simulink model "Appl_VentAdj_CtrlModel"  (R2018b)
settings: configuration reference "CodeConfig_10_ms" (kept outside this file)
undefined symbols (not defined in the file): D_VENT_LVL_1_PRECENT, D_VENT_LVL_2_PRECENT, D_VENT_LVL_3_PRECENT, FALSE, TRUE
libraries: DareLib x72, simulink x1
(part 1 of 4)
settings Model: Creator=Administrator  LastModifiedBy=Administrator
settings ConfigSetRef: SourceLocation=Base Workspace

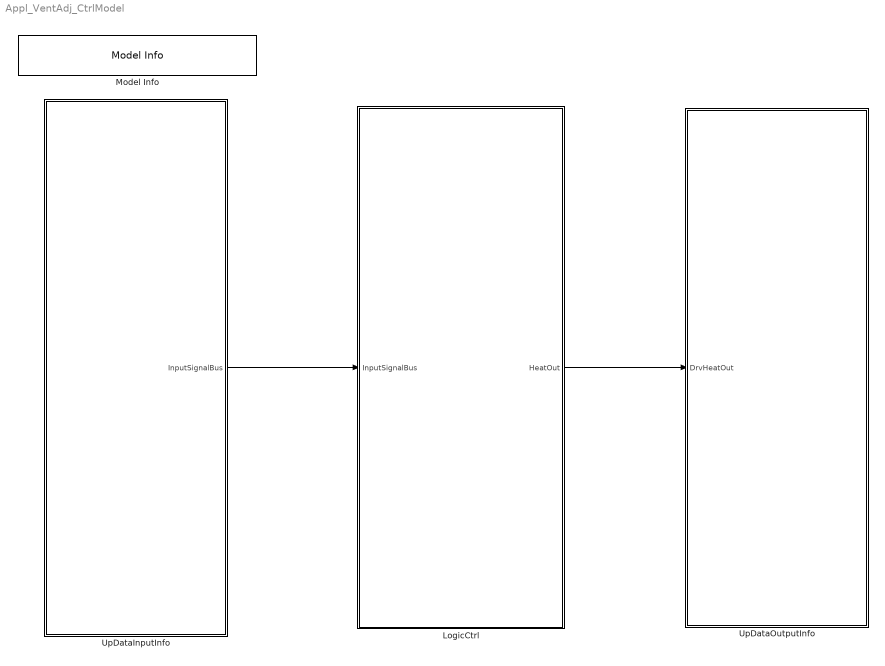
== system Appl_VentAdj_CtrlModel ==
  LogicCtrl : Subsystem  Priority=2  TreatAsAtomicUnit=on
      settings: RTWSystemCode=Nonreusable function  RTWFcnNameOpts=Use subsystem name
  Model Info : simulink/Model-Wide Utilities/Model Info  Frame=on  DisplayStringWithTags=Version：%<ModelVersion>  HorizontalTextAlignment=Center  LeftAlignmentValue=0.5
  UpDataInputInfo : Subsystem  Priority=1  TreatAsAtomicUnit=on
      settings: RTWSystemCode=Nonreusable function  RTWFcnNameOpts=Use subsystem name
  UpDataOutputInfo : Subsystem  Priority=3  TreatAsAtomicUnit=on
      settings: RTWSystemCode=Nonreusable function  RTWFcnNameOpts=Use subsystem name
  wires:
  LogicCtrl/1(HeatOut) -> UpDataOutputInfo/1(DrvHeatOut)
  UpDataInputInfo/1(InputSignalBus) -> LogicCtrl/1(InputSignalBus)

== system Appl_VentAdj_CtrlModel/LogicCtrl ==
  InputSignalBus : Inport
  Bus Selector : BusSelector  OutputSignals=VentRunMaxTime,HeatValid,Rte_SignalBUs.VentAdj_D_SimuIndex_DRVent,Rte_SignalBUs.VentAdj_D_SimuIndex_PAVent,Rte_SignalBUs.VentAdj_D_SimuIndex_ThirdVent,Rte_SignalBUs.VentAdj_CarType,Rte_SignalBUs.VentAdj_RemoteModeFlag,Rte_SignalBUs.VentAdj_EngineRunFlag,Rte_SignalBUs.VentAdj_DriverCmdFaultSts,Rte_SignalBUs.VentAdj_PasCmdFaultSts,Rte_SignalBUs.VentAdj_ThirdCmdFaultSts,Rte_SignalBUs.VentAdj_PowerMode,Rte_SignalBUs.VentAdj_DriverEnableConfig,Rte_SignalBUs.VentAdj_DriverHMI_VentMessage,Rte_SignalBUs.VentAdj_DriverTbox_VentMessage,Rte_SignalBUs.VentAdj_PassengerEnableConfig,Rte_SignalBUs.VentAdj_PassengerHMI_VentMessage,Rte_SignalBUs.VentAdj_PassengerTbox_VentMessage,Rte_SignalBUs.VentAdj_ThirdEnableConfig,Rte_SignalBUs.VentAdj_ThirdHMI_VentMessage,Rte_SignalBUs.VentAdj_ThirdTbox_VentMessage,Rte_SignalBUs.VentAdj_DriverDiagCmd,Rte_SignalBUs.VentAdj_PassengerDiagCmd,Rte_SignalBUs.VentAdj_ThirdDiagCmd,Rte_SignalBUs.VentAdj_TimeOutPrm,Rte_SignalBUs.VentAdj_RunMaxTime,Rte_SignalBUs.VentAdj_VoltMode,Rte_SignalBUs.VentAdj_RecoverDefaultFlag,Rte_SignalBUs.VentAdj_Driver_HMI_HeatMsg,Rte_SignalBUs.VentAdj_Driver_Tbox_HeatMsg,Rte_SignalBUs.VentAdj_Passenger_HMI_HeatMsg,Rte_SignalBUs.VentAdj_Passenger_Tbox_HeatMsg,Rte_SignalBUs.VentAdj_Third_HMI_HeatMsg,Rte_SignalBUs.VentAdj_Third_Tbox_HeatMsg,Rte_SignalBUs.VentAdj_DrVentStopReason,Rte_SignalBUs.VentAdj_PaVentStopReason,Rte_SignalBUs.VentAdj_ThirdVentStopReason,Rte_SignalBUs.VentAdj_VentMsgLostFlag,VentMessage,Rte_SignalBUs.VentAdj_CanDrvVentLvl,Rte_SignalBUs.VentAdj_CanPasVentLvl,Rte_SignalBUs.VentAdj_CanThirdVentLvl,Rte_SignalBUs.VentAdj_DriverCmdFaultSts4DTC,Rte_SignalBUs.VentAdj_PasCmdFaultSts4DTC,Rte_SignalBUs.VentAdj_ThirdCmdFaultSts4DTC,ComPCSatisfiedFlag,VentEnable
  LocalAdjustCtrl : Subsystem  Description=逻辑处理
      settings: AttributesFormatString=%<Description>
  MainVent_OutputLvlSts : BusCreator  Inputs=18
  HeatOut : Outport
  wires:
  InputSignalBus/1 -> Bus Selector/1  "InputSignalBus"
  MainVent_OutputLvlSts/1 -> HeatOut/1
  Bus Selector/1 -> LocalAdjustCtrl/1(VentRunMaxTime)  "<VentRunMaxTime>"
  Bus Selector/2 -> LocalAdjustCtrl/2(HeatValid)  "<HeatValid>"
  Bus Selector/3 -> LocalAdjustCtrl/3(VentAdj_D_SimuIndex_DRVent)  "<VentAdj_D_SimuIndex_DRVent>"
  Bus Selector/4 -> LocalAdjustCtrl/4(VentAdj_D_SimuIndex_PAVent)  "<VentAdj_D_SimuIndex_PAVent>"
  Bus Selector/5 -> LocalAdjustCtrl/5(VentAdj_D_SimuIndex_ThirdVent)  "<VentAdj_D_SimuIndex_ThirdVent>"
  Bus Selector/6 -> LocalAdjustCtrl/6(VentAdj_CarType)  "<VentAdj_CarType>"
  Bus Selector/7 -> LocalAdjustCtrl/7(VentAdj_RemoteModeFlag)  "<VentAdj_RemoteModeFlag>"
  Bus Selector/8 -> LocalAdjustCtrl/8(VentAdj_EngineRunFlag)  "<VentAdj_EngineRunFlag>"
  Bus Selector/9 -> LocalAdjustCtrl/9(VentAdj_DriverCmdFaultSts)  "<VentAdj_DriverCmdFaultSts>"
  Bus Selector/10 -> LocalAdjustCtrl/10(VentAdj_PasCmdFaultSts)  "<VentAdj_PasCmdFaultSts>"
  Bus Selector/11 -> LocalAdjustCtrl/11(VentAdj_ThirdCmdFaultSts)  "<VentAdj_ThirdCmdFaultSts>"
  Bus Selector/12 -> LocalAdjustCtrl/12(VentAdj_PowerMode)  "<VentAdj_PowerMode>"
  Bus Selector/13 -> LocalAdjustCtrl/13(VentAdj_DriverEnableConfig)  "<VentAdj_DriverEnableConfig>"
  Bus Selector/14 -> LocalAdjustCtrl/14(VentAdj_DriverHMI_VentMessage)  "<VentAdj_DriverHMI_VentMessage>"
  Bus Selector/15 -> LocalAdjustCtrl/15(VentAdj_DriverTbox_VentMessage)  "<VentAdj_DriverTbox_VentMessage>"
  Bus Selector/16 -> LocalAdjustCtrl/16(VentAdj_PassengerEnableConfig)  "<VentAdj_PassengerEnableConfig>"
  Bus Selector/17 -> LocalAdjustCtrl/17(VentAdj_PassengerHMI_VentMessage)  "<VentAdj_PassengerHMI_VentMessage>"
  Bus Selector/18 -> LocalAdjustCtrl/18(VentAdj_PassengerTbox_VentMessage)  "<VentAdj_PassengerTbox_VentMessage>"
  Bus Selector/19 -> LocalAdjustCtrl/19(VentAdj_ThirdEnableConfig)  "<VentAdj_ThirdEnableConfig>"
  Bus Selector/20 -> LocalAdjustCtrl/20(VentAdj_ThirdHMI_VentMessage)  "<VentAdj_ThirdHMI_VentMessage>"
  Bus Selector/21 -> LocalAdjustCtrl/21(VentAdj_ThirdTbox_VentMessage)  "<VentAdj_ThirdTbox_VentMessage>"
  Bus Selector/22 -> LocalAdjustCtrl/22(VentAdj_DriverDiagCmd)  "<VentAdj_DriverDiagCmd>"
  Bus Selector/23 -> LocalAdjustCtrl/23(VentAdj_PassengerDiagCmd)  "<VentAdj_PassengerDiagCmd>"
  Bus Selector/24 -> LocalAdjustCtrl/24(VentAdj_ThirdDiagCmd)  "<VentAdj_ThirdDiagCmd>"
  Bus Selector/25 -> LocalAdjustCtrl/25(VentAdj_TimeOutPrm)  "<VentAdj_TimeOutPrm>"
  Bus Selector/26 -> LocalAdjustCtrl/26(VentAdj_RunMaxTime)  "<VentAdj_RunMaxTime>"
  Bus Selector/27 -> LocalAdjustCtrl/27(VentAdj_VoltMode)  "<VentAdj_VoltMode>"
  Bus Selector/28 -> LocalAdjustCtrl/28(VentAdj_RecoverDefaultFlag)  "<VentAdj_RecoverDefaultFlag>"
  Bus Selector/29 -> LocalAdjustCtrl/29(VentAdj_Driver_HMI_HeatMsg)  "<VentAdj_Driver_HMI_HeatMsg>"
  Bus Selector/30 -> LocalAdjustCtrl/30(VentAdj_Driver_Tbox_HeatMsg)  "<VentAdj_Driver_Tbox_HeatMsg>"
  Bus Selector/31 -> LocalAdjustCtrl/31(VentAdj_Passenger_HMI_HeatMsg)  "<VentAdj_Passenger_HMI_HeatMsg>"
  Bus Selector/32 -> LocalAdjustCtrl/32(VentAdj_Passenger_Tbox_HeatMsg)  "<VentAdj_Passenger_Tbox_HeatMsg>"
  Bus Selector/33 -> LocalAdjustCtrl/33(VentAdj_Third_HMI_HeatMsg)  "<VentAdj_Third_HMI_HeatMsg>"
  Bus Selector/34 -> LocalAdjustCtrl/34(VentAdj_Third_Tbox_HeatMsg)  "<VentAdj_Third_Tbox_HeatMsg>"
  Bus Selector/35 -> LocalAdjustCtrl/35(VentAdj_DrVentStopReason)  "<VentAdj_DrVentStopReason>"
  Bus Selector/36 -> LocalAdjustCtrl/36(VentAdj_PaVentStopReason)  "<VentAdj_PaVentStopReason>"
  Bus Selector/37 -> LocalAdjustCtrl/37(VentAdj_ThirdVentStopReason)  "<VentAdj_ThirdVentStopReason>"
  Bus Selector/38 -> LocalAdjustCtrl/38(VentAdj_VentMsgLostFlag)  "<VentAdj_VentMsgLostFlag>"
  LocalAdjustCtrl/1(VentAdj_DrVentStopReasonOut) -> MainVent_OutputLvlSts/1
  LocalAdjustCtrl/2(VentAdj_PaVentStopReasonOut) -> MainVent_OutputLvlSts/2
  LocalAdjustCtrl/3(VentAdj_ThirdVentStopReasonOut) -> MainVent_OutputLvlSts/3
  LocalAdjustCtrl/4(VentAdj_DrVentTypeOut) -> MainVent_OutputLvlSts/4
  LocalAdjustCtrl/5(VentAdj_PaVentTypeOut) -> MainVent_OutputLvlSts/5
  LocalAdjustCtrl/6(VentAdj_ThirdVentTypeOut) -> MainVent_OutputLvlSts/6
  LocalAdjustCtrl/7(HeatAdj_DRVentOut) -> MainVent_OutputLvlSts/7
  LocalAdjustCtrl/8(HeatAdj_PAVentOut) -> MainVent_OutputLvlSts/8
  LocalAdjustCtrl/9(HeatAdj_ThirdVentOut) -> MainVent_OutputLvlSts/9
  LocalAdjustCtrl/10(HeatAdj_DRVentDuty) -> MainVent_OutputLvlSts/10
  LocalAdjustCtrl/11(HeatAdj_PAVentDuty) -> MainVent_OutputLvlSts/11
  LocalAdjustCtrl/12(HeatAdj_ThirdVentDuty) -> MainVent_OutputLvlSts/12
  LocalAdjustCtrl/13(HeatAdj_DrRunStateOut) -> MainVent_OutputLvlSts/13
  LocalAdjustCtrl/14(HeatAdj_PaRunStateOut) -> MainVent_OutputLvlSts/14
  LocalAdjustCtrl/15(HeatAdj_3rdRunStateOut) -> MainVent_OutputLvlSts/15
  Bus Selector/39 -> LocalAdjustCtrl/39(VentMessage)  "<VentMessage>"
  LocalAdjustCtrl/16(DiagDrVentLevel) -> MainVent_OutputLvlSts/16
  LocalAdjustCtrl/17(DiagPaVentLevel) -> MainVent_OutputLvlSts/17
  LocalAdjustCtrl/18(Diag3rdVentLevel) -> MainVent_OutputLvlSts/18
  Bus Selector/40 -> LocalAdjustCtrl/40(VentAdj_CanDrvVentLvl)  "<VentAdj_CanDrvVentLvl>"
  Bus Selector/41 -> LocalAdjustCtrl/41(VentAdj_CanPasVentLvl)  "<VentAdj_CanPasVentLvl>"
  Bus Selector/42 -> LocalAdjustCtrl/42(VentAdj_CanThirdVentLvl)  "<VentAdj_CanThirdVentLvl>"
  Bus Selector/43 -> LocalAdjustCtrl/43(VentAdj_DriverCmdFaultSts4DTC)  "<VentAdj_DriverCmdFaultSts4DTC>"
  Bus Selector/44 -> LocalAdjustCtrl/44(VentAdj_PasCmdFaultSts4DTC)  "<VentAdj_PasCmdFaultSts4DTC>"
  Bus Selector/45 -> LocalAdjustCtrl/45(VentAdj_ThirdCmdFaultSts4DTC)  "<VentAdj_ThirdCmdFaultSts4DTC>"
  Bus Selector/46 -> LocalAdjustCtrl/46(ComPCSatisfiedFlag)  "<ComPCSatisfiedFlag>"
  Bus Selector/47 -> LocalAdjustCtrl/47(VentEnable)  "<VentEnable>"

== system Appl_VentAdj_CtrlModel/UpDataInputInfo ==
  InputSignalProcess : Subsystem  Description=数据处理
      settings: AttributesFormatString=%<Description>  RTWSystemCode=Nonreusable function  RTWFcnNameOpts=Use subsystem name
  RTE : Subsystem  Description=接口自动生成  TreatAsAtomicUnit=on
      settings: AttributesFormatString=%<Description>  RTWSystemCode=Nonreusable function  RTWFcnNameOpts=Use subsystem name
  InputSignalBus : Outport
  wires:
  RTE/1(RTE_Signal) -> InputSignalProcess/1(Rte_SignalBUs)
  InputSignalProcess/1(InputSignalBus) -> InputSignalBus/1

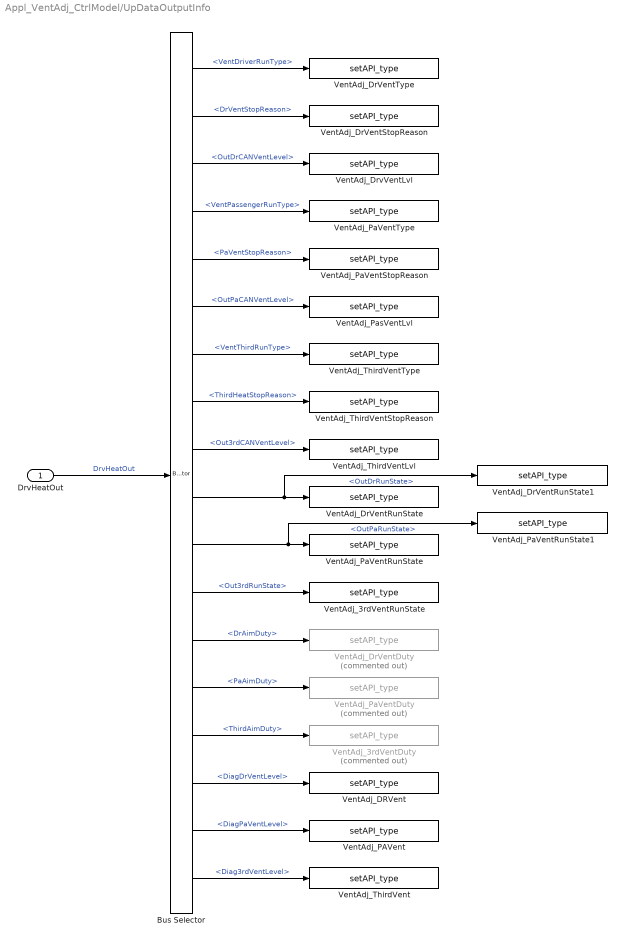
== system Appl_VentAdj_CtrlModel/UpDataOutputInfo ==
  DrvHeatOut : Inport
  Bus Selector : BusSelector  OutputSignals=VentDriverRunType,DrVentStopReason,OutDrCANVentLevel,VentPassengerRunType,PaVentStopReason,OutPaCANVentLevel,VentThirdRunType,ThirdHeatStopReason,Out3rdCANVentLevel,OutDrRunState,OutPaRunState,Out3rdRunState,DrAimDuty,PaAimDuty,ThirdAimDuty,DiagDrVentLevel,DiagPaVentLevel,Diag3rdVentLevel
  VentAdj_3rdVentDuty : DareLib/Dare/setAPI_type  Commented=on  g_funcname=Ecual_PWM_ChannelSetDuty  g_param=""  g_type=uint8  g_size=-1
      settings: AttributesFormatString=%<g_funcname>  SourceProductName=Dare Library
  VentAdj_3rdVentRunState : DareLib/Dare/setAPI_type  g_funcname=Rte_SetVfb_ThirdVentRunState  g_param=""  g_type=uint8  g_size=-1
      settings: AttributesFormatString=%<g_funcname>  SourceProductName=Dare Library
  VentAdj_DRVent : DareLib/Dare/setAPI_type  g_funcname=Rte_SetVfb_DrVent  g_param=""  g_type=uint8  g_enum=enVentLvlSts  g_size=-1
      settings: AttributesFormatString=%<g_funcname>  SourceProductName=Dare Library
  VentAdj_DrVentDuty : DareLib/Dare/setAPI_type  Commented=on  g_funcname=Ecual_PWM_ChannelSetDuty  g_param=""  g_type=uint8  g_size=-1
      settings: AttributesFormatString=%<g_funcname>  SourceProductName=Dare Library
  VentAdj_DrVentRunState : DareLib/Dare/setAPI_type  g_funcname=Rte_SetVfb_DrVentRunState  g_param=""  g_type=uint8  g_size=-1
      settings: AttributesFormatString=%<g_funcname>  SourceProductName=Dare Library
  VentAdj_DrVentRunState1 : DareLib/Dare/setAPI_type  g_funcname=Ecual_CanSetDrvVentSts  g_param=""  g_type=uint8  g_size=-1
      settings: AttributesFormatString=%<g_funcname>  SourceProductName=Dare Library
  VentAdj_DrVentStopReason : DareLib/Dare/setAPI_type  g_funcname=Rte_SetVfb_DrVentStopReason  g_param=""  g_type=uint8  g_enum=enVentStopReason  g_size=-1
      settings: AttributesFormatString=%<g_funcname>  SourceProductName=Dare Library
  VentAdj_DrVentType : DareLib/Dare/setAPI_type  g_funcname=Rte_SetVfb_DrVentType  g_param=""  g_type=uint8  g_enum=enVentType  g_size=-1
      settings: AttributesFormatString=%<g_funcname>  SourceProductName=Dare Library
  VentAdj_DrvVentLvl : DareLib/Dare/setAPI_type  g_funcname=Ecual_CanSetDrvVentLvl  g_param=""  g_type=uint8  g_enum=enVentLvlSts  g_size=-1
      settings: AttributesFormatString=%<g_funcname>  SourceProductName=Dare Library
  VentAdj_PAVent : DareLib/Dare/setAPI_type  g_funcname=Rte_SetVfb_PaVent  g_param=""  g_type=uint8  g_enum=enVentLvlSts  g_size=-1
      settings: AttributesFormatString=%<g_funcname>  SourceProductName=Dare Library
  VentAdj_PaVentDuty : DareLib/Dare/setAPI_type  Commented=on  g_funcname=Ecual_PWM_ChannelSetDuty  g_param=""  g_type=uint8  g_size=-1
      settings: AttributesFormatString=%<g_funcname>  SourceProductName=Dare Library
  VentAdj_PaVentRunState : DareLib/Dare/setAPI_type  g_funcname=Rte_SetVfb_PaVentRunState  g_param=""  g_type=uint8  g_size=-1
      settings: AttributesFormatString=%<g_funcname>  SourceProductName=Dare Library
  VentAdj_PaVentRunState1 : DareLib/Dare/setAPI_type  g_funcname=Ecual_CanSetPasVentSts  g_param=""  g_type=uint8  g_size=-1
      settings: AttributesFormatString=%<g_funcname>  SourceProductName=Dare Library
  VentAdj_PaVentStopReason : DareLib/Dare/setAPI_type  g_funcname=Rte_SetVfb_PaVentStopReason  g_param=""  g_type=uint8  g_enum=enVentStopReason  g_size=-1
      settings: AttributesFormatString=%<g_funcname>  SourceProductName=Dare Library
  VentAdj_PaVentType : DareLib/Dare/setAPI_type  g_funcname=Rte_SetVfb_PaVentType  g_param=""  g_type=uint8  g_enum=enVentType  g_size=-1
      settings: AttributesFormatString=%<g_funcname>  SourceProductName=Dare Library
  VentAdj_PasVentLvl : DareLib/Dare/setAPI_type  g_funcname=Ecual_CanSetPasVentLvl  g_param=""  g_type=uint8  g_enum=enVentLvlSts  g_size=-1
      settings: AttributesFormatString=%<g_funcname>  SourceProductName=Dare Library
  VentAdj_ThirdVent : DareLib/Dare/setAPI_type  g_funcname=Rte_SetVfb_ThirdVent  g_param=""  g_type=uint8  g_enum=enVentLvlSts  g_size=-1
      settings: AttributesFormatString=%<g_funcname>  SourceProductName=Dare Library
  VentAdj_ThirdVentLvl : DareLib/Dare/setAPI_type  g_funcname=Ecual_CanSetThirdVentLvl  g_param=""  g_type=uint8  g_enum=enVentLvlSts  g_size=-1
      settings: AttributesFormatString=%<g_funcname>  SourceProductName=Dare Library
  VentAdj_ThirdVentStopReason : DareLib/Dare/setAPI_type  g_funcname=Rte_SetVfb_ThirdVentStopReason  g_param=""  g_type=uint8  g_enum=enVentStopReason  g_size=-1
      settings: AttributesFormatString=%<g_funcname>  SourceProductName=Dare Library
  VentAdj_ThirdVentType : DareLib/Dare/setAPI_type  g_funcname=Rte_SetVfb_ThirdVentType  g_param=""  g_type=uint8  g_enum=enVentType  g_size=-1
      settings: AttributesFormatString=%<g_funcname>  SourceProductName=Dare Library
  wires:
  DrvHeatOut/1 -> Bus Selector/1  "DrvHeatOut"
  Bus Selector/1 -> VentAdj_DrVentType/1  "<VentDriverRunType>"
  Bus Selector/2 -> VentAdj_DrVentStopReason/1  "<DrVentStopReason>"
  Bus Selector/3 -> VentAdj_DrvVentLvl/1  "<OutDrCANVentLevel>"
  Bus Selector/6 -> VentAdj_PasVentLvl/1  "<OutPaCANVentLevel>"
  Bus Selector/5 -> VentAdj_PaVentStopReason/1  "<PaVentStopReason>"
  Bus Selector/4 -> VentAdj_PaVentType/1  "<VentPassengerRunType>"
  Bus Selector/9 -> VentAdj_ThirdVentLvl/1  "<Out3rdCANVentLevel>"
  Bus Selector/8 -> VentAdj_ThirdVentStopReason/1  "<ThirdHeatStopReason>"
  Bus Selector/7 -> VentAdj_ThirdVentType/1  "<VentThirdRunType>"
  Bus Selector/15 -> VentAdj_3rdVentDuty/1  "<ThirdAimDuty>"
  Bus Selector/14 -> VentAdj_PaVentDuty/1  "<PaAimDuty>"
  Bus Selector/13 -> VentAdj_DrVentDuty/1  "<DrAimDuty>"
  Bus Selector/12 -> VentAdj_3rdVentRunState/1  "<Out3rdRunState>"
  Bus Selector/11 -> VentAdj_PaVentRunState1/1, VentAdj_PaVentRunState/1  "<OutPaRunState>"
  Bus Selector/10 -> VentAdj_DrVentRunState1/1, VentAdj_DrVentRunState/1  "<OutDrRunState>"
  Bus Selector/16 -> VentAdj_DRVent/1  "<DiagDrVentLevel>"
  Bus Selector/17 -> VentAdj_PAVent/1  "<DiagPaVentLevel>"
  Bus Selector/18 -> VentAdj_ThirdVent/1  "<Diag3rdVentLevel>"

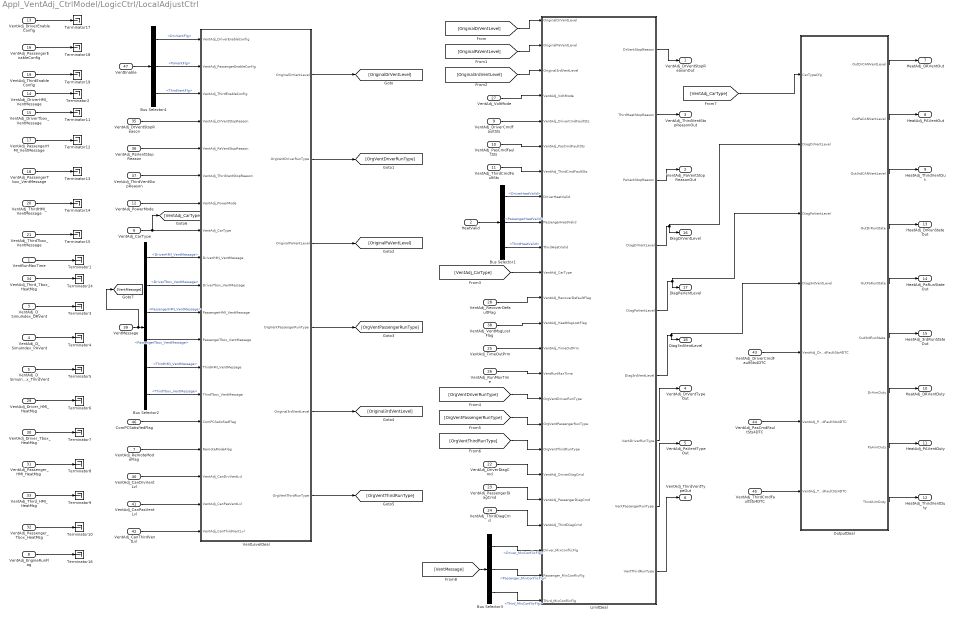
== system Appl_VentAdj_CtrlModel/LogicCtrl/LocalAdjustCtrl ==
  VentRunMaxTime : Inport
  HeatValid : Inport  Port=2
  VentAdj_D_SimuIndex_DRVent : Inport  Port=3
  VentAdj_D_SimuIndex_PAVent : Inport  Port=4
  VentAdj_D_SimuIndex_ThirdVent : Inport  Port=5
  VentAdj_CarType : Inport  Port=6
  VentAdj_RemoteModeFlag : Inport  Port=7
  VentAdj_EngineRunFlag : Inport  Port=8
  VentAdj_DriverCmdFaultSts : Inport  Port=9
  VentAdj_PasCmdFaultSts : Inport  Port=10
  VentAdj_ThirdCmdFaultSts : Inport  Port=11
  VentAdj_PowerMode : Inport  Port=12
  VentAdj_DriverEnableConfig : Inport  Port=13
  VentAdj_DriverHMI_VentMessage : Inport  Port=14
  VentAdj_DriverTbox_VentMessage : Inport  Port=15
  VentAdj_PassengerEnableConfig : Inport  Port=16
  VentAdj_PassengerHMI_VentMessage : Inport  Port=17
  VentAdj_PassengerTbox_VentMessage : Inport  Port=18
  VentAdj_ThirdEnableConfig : Inport  Port=19
  VentAdj_ThirdHMI_VentMessage : Inport  Port=20
  VentAdj_ThirdTbox_VentMessage : Inport  Port=21
  VentAdj_DriverDiagCmd : Inport  Port=22
  VentAdj_PassengerDiagCmd : Inport  Port=23
  VentAdj_ThirdDiagCmd : Inport  Port=24
  VentAdj_TimeOutPrm : Inport  Port=25
  VentAdj_RunMaxTime : Inport  Port=26
  VentAdj_VoltMode : Inport  Port=27
  VentAdj_RecoverDefaultFlag : Inport  Port=28
  VentAdj_Driver_HMI_HeatMsg : Inport  Port=29
  VentAdj_Driver_Tbox_HeatMsg : Inport  Port=30
  VentAdj_Passenger_HMI_HeatMsg : Inport  Port=31
  VentAdj_Passenger_Tbox_HeatMsg : Inport  Port=32
  VentAdj_Third_HMI_HeatMsg : Inport  Port=33
  VentAdj_Third_Tbox_HeatMsg : Inport  Port=34
  VentAdj_DrVentStopReason : Inport  Port=35
  VentAdj_PaVentStopReason : Inport  Port=36
  VentAdj_ThirdVentStopReason : Inport  Port=37
  VentAdj_VentMsgLostFlag : Inport  Port=38
  VentMessage : Inport  Port=39
  VentAdj_CanDrvVentLvl : Inport  Port=40
  VentAdj_CanPasVentLvl : Inport  Port=41
  VentAdj_CanThirdVentLvl : Inport  Port=42
  VentAdj_DriverCmdFaultSts4DTC : Inport  Port=43
  VentAdj_PasCmdFaultSts4DTC : Inport  Port=44
  VentAdj_ThirdCmdFaultSts4DTC : Inport  Port=45
  ComPCSatisfiedFlag : Inport  Port=46
  VentEnable : Inport  Port=47
  Bus Selector1 : BusSelector  OutputSignals=DriverHeatValid,PassengerHeatValid,ThirdHeatValid
  Bus Selector2 : BusSelector  OutputSignals=DriverHMI_VentMessage,DriverTbox_VentMessage,PassengerHMI_VentMessage,PassengerTbox_VentMessage,ThirdHMI_VentMessage,ThirdTbox_VentMessage
  Bus Selector3 : BusSelector  OutputSignals=Driver_MixConflicFlg,Passenger_MixConflicFlg,Third_MixConflicFlg
  Bus Selector4 : BusSelector  OutputSignals=DrvVentFlg,PaVentFlg,ThirdVentFlg
  LimitDeal : Stateflow chart  TreatAsAtomicUnit=on
  OutputDeal : Stateflow chart  TreatAsAtomicUnit=on
  Terminator{1..19,24} (20 alike) : Terminator
  VentLevelDeal : Stateflow chart  TreatAsAtomicUnit=on
  VentAdj_DrVentStopReasonOut : Outport
  VentAdj_PaVentStopReasonOut : Outport  Port=2
  VentAdj_ThirdVentStopReasonOut : Outport  Port=3
  VentAdj_DrVentTypeOut : Outport  Port=4
  VentAdj_PaVentTypeOut : Outport  Port=5
  VentAdj_ThirdVentTypeOut : Outport  Port=6
  HeatAdj_DRVentOut : Outport  Port=7
  HeatAdj_PAVentOut : Outport  Port=8
  HeatAdj_ThirdVentOut : Outport  Port=9
  HeatAdj_DRVentDuty : Outport  Port=10
  HeatAdj_PAVentDuty : Outport  Port=11
  HeatAdj_ThirdVentDuty : Outport  Port=12
  HeatAdj_DrRunStateOut : Outport  Port=13
  HeatAdj_PaRunStateOut : Outport  Port=14
  HeatAdj_3rdRunStateOut : Outport  Port=15
  DiagDrVentLevel : Outport  Port=16
  DiagPaVentLevel : Outport  Port=17
  Diag3rdVentLevel : Outport  Port=18
  wires:
  VentLevelDeal/1(OriginalDrVentLevel) -> [OriginalDrVentLevel]
  VentLevelDeal/2(OrgVentDriverRunType) -> [OrgVentDriverRunType]
  VentLevelDeal/3(OriginalPaVentLevel) -> [OriginalPaVentLevel]
  VentLevelDeal/4(OrgVentPassengerRunType) -> [OrgVentPassengerRunType]
  VentLevelDeal/5(Original3rdVentLevel) -> [Original3rdVentLevel]
  VentLevelDeal/6(OrgVentThirdRunType) -> [OrgVentThirdRunType]
  LimitDeal/1(DrVentStopReason) -> VentAdj_DrVentStopReasonOut/1
  LimitDeal/3(PaVentStopReason) -> VentAdj_PaVentStopReasonOut/1
  LimitDeal/2(ThirdHeatStopReason) -> VentAdj_ThirdVentStopReasonOut/1
  LimitDeal/7(VentDriverRunType) -> VentAdj_DrVentTypeOut/1
  LimitDeal/8(VentPassengerRunType) -> VentAdj_PaVentTypeOut/1
  LimitDeal/9(VentThirdRunType) -> VentAdj_ThirdVentTypeOut/1
  OutputDeal/1(OutDrCANVentLevel) -> HeatAdj_DRVentOut/1
  OutputDeal/2(OutPaCANVentLevel) -> HeatAdj_PAVentOut/1
  OutputDeal/3(Out3rdCANVentLevel) -> HeatAdj_ThirdVentOut/1
  OutputDeal/4(OutDrRunState) -> HeatAdj_DrRunStateOut/1
  OutputDeal/5(OutPaRunState) -> HeatAdj_PaRunStateOut/1
  OutputDeal/6(Out3rdRunState) -> HeatAdj_3rdRunStateOut/1
  HeatValid/1 -> Bus Selector1/1
  VentRunMaxTime/1 -> Terminator1/1
  VentAdj_Third_Tbox_HeatMsg/1 -> Terminator24/1
  VentAdj_D_SimuIndex_DRVent/1 -> Terminator3/1
  VentAdj_D_SimuIndex_ThirdVent/1 -> Terminator5/1
  VentAdj_D_SimuIndex_PAVent/1 -> Terminator4/1
  VentAdj_Driver_HMI_HeatMsg/1 -> Terminator6/1
  VentAdj_Driver_Tbox_HeatMsg/1 -> Terminator7/1
  VentAdj_Passenger_HMI_HeatMsg/1 -> Terminator8/1
  VentAdj_Third_HMI_HeatMsg/1 -> Terminator9/1
  VentAdj_Passenger_Tbox_HeatMsg/1 -> Terminator10/1
  VentAdj_DrVentStopReason/1 -> VentLevelDeal/4(VentAdj_DrVentStopReason)
  VentAdj_PaVentStopReason/1 -> VentLevelDeal/5(VentAdj_PaVentStopReason)
  VentAdj_ThirdVentStopReason/1 -> VentLevelDeal/6(VentAdj_ThirdVentStopReason)
  VentAdj_PowerMode/1 -> VentLevelDeal/7(VentAdj_PowerMode)
  VentAdj_CarType/1 -> VentLevelDeal/8(VentAdj_CarType), [VentAdj_CarType]
  VentAdj_RemoteModeFlag/1 -> VentLevelDeal/16(RemoteModeFlag)
  [OriginalDrVentLevel] -> LimitDeal/1(OriginalDrVentLevel)
  [OriginalPaVentLevel] -> LimitDeal/2(OriginalPaVentLevel)
  [Original3rdVentLevel] -> LimitDeal/3(Original3rdVentLevel)
  VentAdj_VoltMode/1 -> LimitDeal/4(VentAdj_VoltMode)
  VentAdj_DriverCmdFaultSts/1 -> LimitDeal/5(VentAdj_DriverCmdFaultSts)
  VentAdj_PasCmdFaultSts/1 -> LimitDeal/6(VentAdj_PasCmdFaultSts)
  VentAdj_ThirdCmdFaultSts/1 -> LimitDeal/7(VentAdj_ThirdCmdFaultSts)
  Bus Selector1/1 -> LimitDeal/8(DriverHeatValid)  "<DriverHeatValid>"
  Bus Selector1/2 -> LimitDeal/9(PassengerHeatValid)  "<PassengerHeatValid>"
  Bus Selector1/3 -> LimitDeal/10(ThirdHeatValid)  "<ThirdHeatValid>"
  [OrgVentDriverRunType] -> LimitDeal/16(OrgVentDriverRunType)
  [OrgVentPassengerRunType] -> LimitDeal/17(OrgVentPassengerRunType)
  [OrgVentThirdRunType] -> LimitDeal/18(OrgVentThirdRunType)
  [VentAdj_CarType] -> LimitDeal/11(VentAdj_CarType)
  VentAdj_RecoverDefaultFlag/1 -> LimitDeal/12(VentAdj_RecoverDefaultFlag)
  VentAdj_TimeOutPrm/1 -> LimitDeal/14(VentAdj_TimeOutPrm)
  VentAdj_VentMsgLostFlag/1 -> LimitDeal/13(VentAdj_HeatMsgLostFlag)
  VentAdj_RunMaxTime/1 -> LimitDeal/15(VentRunMaxTime)
  VentAdj_DriverDiagCmd/1 -> LimitDeal/19(VentAdj_DriverDiagCmd)
  VentAdj_PassengerDiagCmd/1 -> LimitDeal/20(VentAdj_PassengerDiagCmd)
  VentAdj_ThirdDiagCmd/1 -> LimitDeal/21(VentAdj_ThirdDiagCmd)
  LimitDeal/6(Diag3rdVentLevel) -> OutputDeal/4(Diag3rdVentLevel), Diag3rdVentLevel/1
  LimitDeal/5(DiagPaVentLevel) -> OutputDeal/3(DiagPaVentLevel), DiagPaVentLevel/1
  LimitDeal/4(DiagDrVentLevel) -> OutputDeal/2(DiagDrVentLevel), DiagDrVentLevel/1
  [VentAdj_CarType] -> OutputDeal/1(CarTypeCfg)
  OutputDeal/9(ThirdAimDuty) -> HeatAdj_ThirdVentDuty/1
  OutputDeal/8(PaAimDuty) -> HeatAdj_PAVentDuty/1
  OutputDeal/7(DrAimDuty) -> HeatAdj_DRVentDuty/1
  VentMessage/1 -> [VentMessage], Bus Selector2/1
  Bus Selector2/1 -> VentLevelDeal/9(DriverHMI_VentMessage)  "<DriverHMI_VentMessage>"
  Bus Selector2/2 -> VentLevelDeal/10(DriverTbox_VentMessage)  "<DriverTbox_VentMessage>"
  Bus Selector2/3 -> VentLevelDeal/11(PassengerHMI_VentMessage)  "<PassengerHMI_VentMessage>"
  Bus Selector2/4 -> VentLevelDeal/12(PassengerTbox_VentMessage)  "<PassengerTbox_VentMessage>"
  Bus Selector2/5 -> VentLevelDeal/13(ThirdHMI_VentMessage)  "<ThirdHMI_VentMessage>"
  Bus Selector2/6 -> VentLevelDeal/14(ThirdTbox_VentMessage)  "<ThirdTbox_VentMessage>"
  VentAdj_PassengerTbox_VentMessage/1 -> Terminator13/1
  VentAdj_ThirdHMI_VentMessage/1 -> Terminator14/1
  VentAdj_PassengerHMI_VentMessage/1 -> Terminator12/1
  VentAdj_DriverTbox_VentMessage/1 -> Terminator11/1
  VentAdj_DriverHMI_VentMessage/1 -> Terminator2/1
  VentAdj_ThirdTbox_VentMessage/1 -> Terminator15/1
  VentAdj_CanDrvVentLvl/1 -> VentLevelDeal/17(VentAdj_CanDrvVentLvl)
  VentAdj_PasCmdFaultSts4DTC/1 -> OutputDeal/6(VentAdj_PasCmdFaultSts4DTC)
  VentAdj_DriverCmdFaultSts4DTC/1 -> OutputDeal/5(VentAdj_DriverCmdFaultSts4DTC)
  VentAdj_ThirdCmdFaultSts4DTC/1 -> OutputDeal/7(VentAdj_ThirdCmdFaultSts4DTC)
  VentAdj_CanPasVentLvl/1 -> VentLevelDeal/18(VentAdj_CanPasVentLvl)
  VentAdj_CanThirdVentLvl/1 -> VentLevelDeal/19(VentAdj_CanThirdVentLvl)
  [VentMessage] -> Bus Selector3/1
  Bus Selector3/1 -> LimitDeal/22(Driver_MixConflicFlg)  "<Driver_MixConflicFlg>"
  Bus Selector3/2 -> LimitDeal/23(Passenger_MixConflicFlg)  "<Passenger_MixConflicFlg>"
  Bus Selector3/3 -> LimitDeal/24(Third_MixConflicFlg)  "<Third_MixConflicFlg>"
  VentAdj_EngineRunFlag/1 -> Terminator16/1
  ComPCSatisfiedFlag/1 -> VentLevelDeal/15(ComPCSatisfiedFlag)
  VentAdj_DriverEnableConfig/1 -> Terminator17/1
  VentAdj_PassengerEnableConfig/1 -> Terminator18/1
  VentAdj_ThirdEnableConfig/1 -> Terminator19/1
  VentEnable/1 -> Bus Selector4/1
  Bus Selector4/3 -> VentLevelDeal/3(VentAdj_ThirdEnableConfig)  "<ThirdVentFlg>"
  Bus Selector4/2 -> VentLevelDeal/2(VentAdj_PassengerEnableConfig)  "<PaVentFlg>"
  Bus Selector4/1 -> VentLevelDeal/1(VentAdj_DriverEnableConfig)  "<DrvVentFlg>"

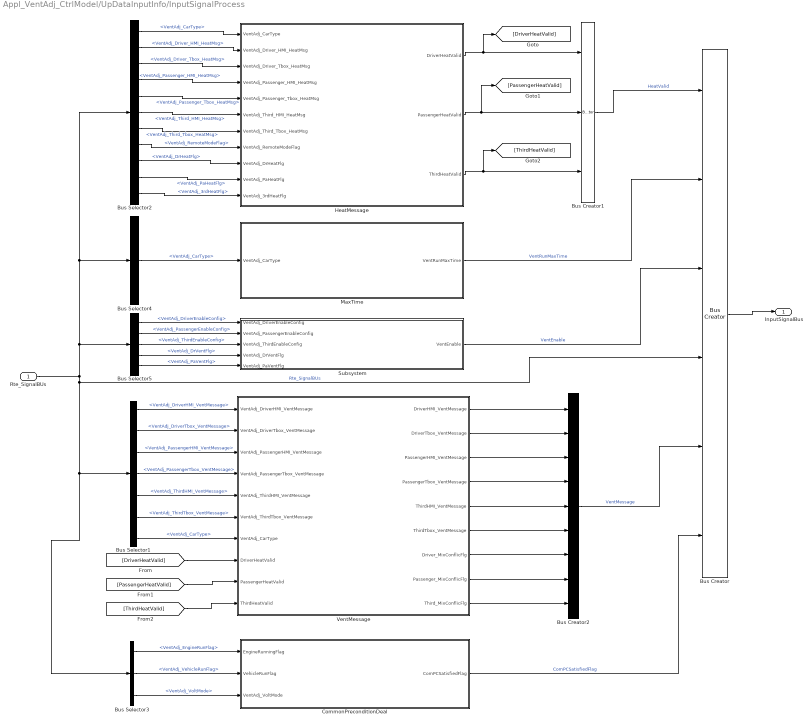
== system Appl_VentAdj_CtrlModel/UpDataInputInfo/InputSignalProcess ==
  Rte_SignalBUs : Inport
  Bus Creator : BusCreator  Inputs=6
  Bus Creator1 : BusCreator  Inputs=3
  Bus Creator2 : BusCreator  Inputs=9
  Bus Selector1 : BusSelector  OutputSignals=VentAdj_DriverHMI_VentMessage,VentAdj_DriverTbox_VentMessage,VentAdj_PassengerHMI_VentMessage,VentAdj_PassengerTbox_VentMessage,VentAdj_ThirdHMI_VentMessage,VentAdj_ThirdTbox_VentMessage,VentAdj_CarType
  Bus Selector2 : BusSelector  OutputSignals=VentAdj_CarType,VentAdj_Driver_HMI_HeatMsg,VentAdj_Driver_Tbox_HeatMsg,VentAdj_Passenger_HMI_HeatMsg,VentAdj_Passenger_Tbox_HeatMsg,VentAdj_Third_HMI_HeatMsg,VentAdj_Third_Tbox_HeatMsg,VentAdj_RemoteModeFlag,VentAdj_DrHeatFlg,VentAdj_PaHeatFlg,VentAdj_3rdHeatFlg
  Bus Selector3 : BusSelector  OutputSignals=VentAdj_EngineRunFlag,VentAdj_VehicleRunFlag,VentAdj_VoltMode
  Bus Selector4 : BusSelector  OutputSignals=VentAdj_CarType
  Bus Selector5 : BusSelector  OutputSignals=VentAdj_DriverEnableConfig,VentAdj_PassengerEnableConfig,VentAdj_ThirdEnableConfig,VentAdj_DrVentFlg,VentAdj_PaVentFlg
  CommonPreconditionDeal : Subsystem  Description=通用前置条件处理
      settings: AttributesFormatString=%<Description>
      mask Display: image('加热通用前置条件.png');
  HeatMessage : Subsystem  Description=加热报文处理
      settings: AttributesFormatString=%<Description>
      mask Display: image('加热报文处理.png');
  MaxTime : Subsystem  Description=最大运行时间
      settings: AttributesFormatString=%<Description>
      mask Display: image('最大运行时间.png');
  Subsystem : Subsystem
  VentMessage : Subsystem  Description=通风报文处理
      settings: AttributesFormatString=%<Description>
      mask Display: image('通风报文处理.png');
  InputSignalBus : Outport
  wires:
  Bus Creator/1 -> InputSignalBus/1
  Rte_SignalBUs/1 -> Bus Selector3/1, Bus Selector1/1, Bus Creator/4, Bus Selector2/1, Bus Selector4/1, Bus Selector5/1  "Rte_SignalBUs"
  Bus Selector2/1 -> HeatMessage/1(VentAdj_CarType)  "<VentAdj_CarType>"
  Bus Selector2/2 -> HeatMessage/2(VentAdj_Driver_HMI_HeatMsg)  "<VentAdj_Driver_HMI_HeatMsg>"
  Bus Selector2/3 -> HeatMessage/3(VentAdj_Driver_Tbox_HeatMsg)  "<VentAdj_Driver_Tbox_HeatMsg>"
  Bus Selector2/4 -> HeatMessage/4(VentAdj_Passenger_HMI_HeatMsg)  "<VentAdj_Passenger_HMI_HeatMsg>"
  Bus Selector2/5 -> HeatMessage/5(VentAdj_Passenger_Tbox_HeatMsg)  "<VentAdj_Passenger_Tbox_HeatMsg>"
  Bus Selector2/6 -> HeatMessage/6(VentAdj_Third_HMI_HeatMsg)  "<VentAdj_Third_HMI_HeatMsg>"
  Bus Selector2/7 -> HeatMessage/7(VentAdj_Third_Tbox_HeatMsg)  "<VentAdj_Third_Tbox_HeatMsg>"
  Bus Selector2/8 -> HeatMessage/8(VentAdj_RemoteModeFlag)  "<VentAdj_RemoteModeFlag>"
  HeatMessage/2(PassengerHeatValid) -> [PassengerHeatValid], Bus Creator1/2
  HeatMessage/3(ThirdHeatValid) -> [ThirdHeatValid], Bus Creator1/3
  HeatMessage/1(DriverHeatValid) -> [DriverHeatValid], Bus Creator1/1
  Bus Selector4/1 -> MaxTime/1(VentAdj_CarType)  "<VentAdj_CarType>"
  MaxTime/1(VentRunMaxTime) -> Bus Creator/2  "VentRunMaxTime"
  Bus Creator1/1 -> Bus Creator/1  "HeatValid"
  Bus Selector1/1 -> VentMessage/1(VentAdj_DriverHMI_VentMessage)  "<VentAdj_DriverHMI_VentMessage>"
  Bus Selector1/2 -> VentMessage/2(VentAdj_DriverTbox_VentMessage)  "<VentAdj_DriverTbox_VentMessage>"
  Bus Selector1/3 -> VentMessage/3(VentAdj_PassengerHMI_VentMessage)  "<VentAdj_PassengerHMI_VentMessage>"
  Bus Selector1/4 -> VentMessage/4(VentAdj_PassengerTbox_VentMessage)  "<VentAdj_PassengerTbox_VentMessage>"
  Bus Selector1/5 -> VentMessage/5(VentAdj_ThirdHMI_VentMessage)  "<VentAdj_ThirdHMI_VentMessage>"
  Bus Selector1/6 -> VentMessage/6(VentAdj_ThirdTbox_VentMessage)  "<VentAdj_ThirdTbox_VentMessage>"
  [DriverHeatValid] -> VentMessage/8(DriverHeatValid)
  [ThirdHeatValid] -> VentMessage/10(ThirdHeatValid)
  [PassengerHeatValid] -> VentMessage/9(PassengerHeatValid)
  VentMessage/1(DriverHMI_VentMessage) -> Bus Creator2/1
  VentMessage/2(DriverTbox_VentMessage) -> Bus Creator2/2
  VentMessage/3(PassengerHMI_VentMessage) -> Bus Creator2/3
  VentMessage/4(PassengerTbox_VentMessage) -> Bus Creator2/4
  VentMessage/5(ThirdHMI_VentMessage) -> Bus Creator2/5
  VentMessage/6(ThirdTbox_VentMessage) -> Bus Creator2/6
  Bus Creator2/1 -> Bus Creator/5  "VentMessage"
  Bus Selector1/7 -> VentMessage/7(VentAdj_CarType)  "<VentAdj_CarType>"
  VentMessage/7(Driver_MixConflicFlg) -> Bus Creator2/7
  VentMessage/8(Passenger_MixConflicFlg) -> Bus Creator2/8
  VentMessage/9(Third_MixConflicFlg) -> Bus Creator2/9
  Bus Selector3/1 -> CommonPreconditionDeal/1(EngineRunningFlag)  "<VentAdj_EngineRunFlag>"
  Bus Selector3/2 -> CommonPreconditionDeal/2(VehicleRunFlag)  "<VentAdj_VehicleRunFlag>"
  CommonPreconditionDeal/1("ComPCSatisfiedFlag ") -> Bus Creator/6  "ComPCSatisfiedFlag"
  Bus Selector3/3 -> CommonPreconditionDeal/3(VentAdj_VoltMode)  "<VentAdj_VoltMode>"
  Bus Selector5/3 -> Subsystem/3(VentAdj_ThirdEnableConfig)  "<VentAdj_ThirdEnableConfig>"
  Bus Selector5/2 -> Subsystem/2(VentAdj_PassengerEnableConfig)  "<VentAdj_PassengerEnableConfig>"
  Bus Selector5/4 -> Subsystem/4(VentAdj_DrVentFlg)  "<VentAdj_DrVentFlg>"
  Bus Selector5/1 -> Subsystem/1(VentAdj_DriverEnableConfig)  "<VentAdj_DriverEnableConfig>"
  Bus Selector5/5 -> Subsystem/5(VentAdj_PaVentFlg)  "<VentAdj_PaVentFlg>"
  Subsystem/1(VentEnable) -> Bus Creator/3  "VentEnable"
  Bus Selector2/9 -> HeatMessage/9(VentAdj_DrHeatFlg)  "<VentAdj_DrHeatFlg>"
  Bus Selector2/10 -> HeatMessage/10(VentAdj_PaHeatFlg)  "<VentAdj_PaHeatFlg>"
  Bus Selector2/11 -> HeatMessage/11(VentAdj_3rdHeatFlg)  "<VentAdj_3rdHeatFlg>"

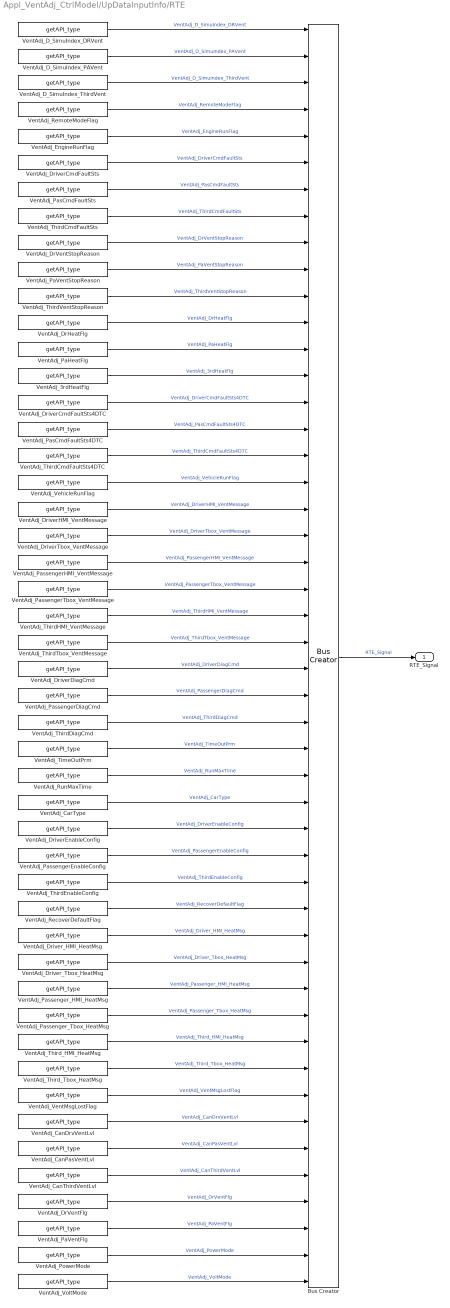
== system Appl_VentAdj_CtrlModel/UpDataInputInfo/RTE ==
  Bus Creator : BusCreator  Inputs=48
  VentAdj_3rdHeatFlg : DareLib/Dare/getAPI_type  g_funcname=Rte_GetVfb_ThirdHeatEnable  g_param=""  g_type=uint8  g_size=-1
      settings: AttributesFormatString=%<g_funcname>  SourceProductName=Dare Library
  VentAdj_CanDrvVentLvl : DareLib/Dare/getAPI_type  g_funcname=Ecual_CanGetDrvVentLvl  g_param=""  g_type=uint8  g_size=-1
      settings: AttributesFormatString=%<g_funcname>  SourceProductName=Dare Library
  VentAdj_CanPasVentLvl : DareLib/Dare/getAPI_type  g_funcname=Ecual_CanGetPasVentLvl  g_param=""  g_type=uint8  g_size=-1
      settings: AttributesFormatString=%<g_funcname>  SourceProductName=Dare Library
  VentAdj_CanThirdVentLvl : DareLib/Dare/getAPI_type  g_funcname=Ecual_CanGetThirdVentLvl  g_param=""  g_type=uint8  g_size=-1
      settings: AttributesFormatString=%<g_funcname>  SourceProductName=Dare Library
  VentAdj_CarType : DareLib/Dare/getAPI_type  g_funcname=Srvl_GetMemIndexDataU8  g_param=EN_MemIndex_Heat_CarType  g_type=uint8  g_enum=enProjectType  g_size=-1
      settings: AttributesFormatString=%<g_funcname>  SourceProductName=Dare Library
  VentAdj_D_SimuIndex_DRVent : DareLib/Dare/getAPI_type  g_funcname=Rte_GetVfb_DrVent  g_param=""  g_type=uint8  g_enum=enVentLvlSts  g_size=-1
      settings: AttributesFormatString=%<g_funcname>  SourceProductName=Dare Library
  VentAdj_D_SimuIndex_PAVent : DareLib/Dare/getAPI_type  g_funcname=Rte_GetVfb_PaVent  g_param=""  g_type=uint8  g_enum=enVentLvlSts  g_size=-1
      settings: AttributesFormatString=%<g_funcname>  SourceProductName=Dare Library
  VentAdj_D_SimuIndex_ThirdVent : DareLib/Dare/getAPI_type  g_funcname=Rte_GetVfb_ThirdVent  g_param=""  g_type=uint8  g_enum=enVentLvlSts  g_size=-1
      settings: AttributesFormatString=%<g_funcname>  SourceProductName=Dare Library
  VentAdj_DrHeatFlg : DareLib/Dare/getAPI_type  g_funcname=Rte_GetVfb_DrHeatEnable  g_param=""  g_type=uint8  g_size=-1
      settings: AttributesFormatString=%<g_funcname>  SourceProductName=Dare Library
  VentAdj_DrVentFlg : DareLib/Dare/getAPI_type  g_funcname=Rte_GetVfb_DrVentEnable  g_param=""  g_type=uint8  g_size=-1
      settings: AttributesFormatString=%<g_funcname>  SourceProductName=Dare Library
  VentAdj_DrVentStopReason : DareLib/Dare/getAPI_type  g_funcname=Rte_GetVfb_DrVentStopReason  g_param=""  g_type=uint8  g_enum=enVentStopReason  g_size=-1
      settings: AttributesFormatString=%<g_funcname>  SourceProductName=Dare Library
  VentAdj_DriverCmdFaultSts : DareLib/Dare/getAPI_type  g_funcname=Rte_GetVfb_DrVentCmdFaultSts  g_param=""  g_type=uint8  g_enum=enVentCmdFault  g_size=-1
      settings: AttributesFormatString=%<g_funcname>  SourceProductName=Dare Library
  VentAdj_DriverCmdFaultSts4DTC : DareLib/Dare/getAPI_type  g_funcname=Rte_GetVfb_DrVentCmdFaultSts4DTC  g_param=""  g_type=uint8  g_enum=enVentCmdFault  g_size=-1
      settings: AttributesFormatString=%<g_funcname>  SourceProductName=Dare Library
  VentAdj_DriverDiagCmd : DareLib/Dare/getAPI_type  g_funcname=Desc_DiagOutCtrlPram  g_param=EN_DRVENTILATE  g_type=uint8  g_enum=enVentIoCmdLvl  g_size=-1
      settings: AttributesFormatString=%<g_funcname>  SourceProductName=Dare Library
  VentAdj_DriverEnableConfig : DareLib/Dare/getAPI_type  g_funcname=Rte_GetVfb_DrVentEnable  g_param=""  g_type=uint8  g_size=-1
      settings: AttributesFormatString=%<g_funcname>  SourceProductName=Dare Library
  VentAdj_DriverHMI_VentMessage : DareLib/Dare/getAPI_type  g_funcname=CanRx_0x351_IVI_FLSeatVentnSet  g_param=""  g_type=uint8  g_size=-1
      settings: AttributesFormatString=%<g_funcname>  SourceProductName=Dare Library
  VentAdj_DriverTbox_VentMessage : DareLib/Dare/getAPI_type  g_funcname=CanRx_0x281_BDC_TBOX_Req_DrSeatVentilating  g_param=""  g_type=uint8  g_size=-1
      settings: AttributesFormatString=%<g_funcname>  SourceProductName=Dare Library
  VentAdj_Driver_HMI_HeatMsg : DareLib/Dare/getAPI_type  g_funcname=CanRx_0x351_IVI_FLSeatHeatSet  g_param=""  g_type=uint8  g_size=-1
      settings: AttributesFormatString=%<g_funcname>  SourceProductName=Dare Library
  VentAdj_Driver_Tbox_HeatMsg : DareLib/Dare/getAPI_type  g_funcname=CanRx_0x281_BDC_TBOX_Req_DrSeatHeating  g_param=""  g_type=uint8  g_size=-1
      settings: AttributesFormatString=%<g_funcname>  SourceProductName=Dare Library
  VentAdj_EngineRunFlag : DareLib/Dare/getAPI_type  g_funcname=Rte_GetVfb_EngineRunFlag  g_param=""  g_type=uint8  g_size=-1
      settings: AttributesFormatString=%<g_funcname>  SourceProductName=Dare Library
  VentAdj_PaHeatFlg : DareLib/Dare/getAPI_type  g_funcname=Rte_GetVfb_SecondHeatEnable  g_param=""  g_type=uint8  g_size=-1
      settings: AttributesFormatString=%<g_funcname>  SourceProductName=Dare Library
  VentAdj_PaVentFlg : DareLib/Dare/getAPI_type  g_funcname=Rte_GetVfb_SecondVentEnable  g_param=""  g_type=uint8  g_size=-1
      settings: AttributesFormatString=%<g_funcname>  SourceProductName=Dare Library
  VentAdj_PaVentStopReason : DareLib/Dare/getAPI_type  g_funcname=Rte_GetVfb_PaVentStopReason  g_param=""  g_type=uint8  g_enum=enVentStopReason  g_size=-1
      settings: AttributesFormatString=%<g_funcname>  SourceProductName=Dare Library
  VentAdj_PasCmdFaultSts : DareLib/Dare/getAPI_type  g_funcname=Rte_GetVfb_PaVentCmdFaultSts  g_param=""  g_type=uint8  g_enum=enVentCmdFault  g_size=-1
      settings: AttributesFormatString=%<g_funcname>  SourceProductName=Dare Library
  VentAdj_PasCmdFaultSts4DTC : DareLib/Dare/getAPI_type  g_funcname=Rte_GetVfb_PaVentCmdFaultSts4DTC  g_param=""  g_type=uint8  g_enum=enVentCmdFault  g_size=-1
      settings: AttributesFormatString=%<g_funcname>  SourceProductName=Dare Library
  VentAdj_PassengerDiagCmd : DareLib/Dare/getAPI_type  g_funcname=Desc_DiagOutCtrlPram  g_param=EN_PAVENTILATE  g_type=uint8  g_enum=enVentIoCmdLvl  g_size=-1
      settings: AttributesFormatString=%<g_funcname>  SourceProductName=Dare Library
  VentAdj_PassengerEnableConfig : DareLib/Dare/getAPI_type  g_funcname=Rte_GetVfb_SecondVentEnable  g_param=""  g_type=uint8  g_size=-1
      settings: AttributesFormatString=%<g_funcname>  SourceProductName=Dare Library
  VentAdj_PassengerHMI_VentMessage : DareLib/Dare/getAPI_type  g_funcname=CanRx_0x351_IVI_FRSeatVentnSet  g_param=""  g_type=uint8  g_size=-1
      settings: AttributesFormatString=%<g_funcname>  SourceProductName=Dare Library
  VentAdj_PassengerTbox_VentMessage : DareLib/Dare/getAPI_type  g_funcname=CanRx_0x281_BDC_TBOX_Req_PaSeatVentilating  g_param=""  g_type=uint8  g_size=-1
      settings: AttributesFormatString=%<g_funcname>  SourceProductName=Dare Library
  VentAdj_Passenger_HMI_HeatMsg : DareLib/Dare/getAPI_type  g_funcname=CanRx_0x351_IVI_FRSeatHeatSet  g_param=""  g_type=uint8  g_size=-1
      settings: AttributesFormatString=%<g_funcname>  SourceProductName=Dare Library
  VentAdj_Passenger_Tbox_HeatMsg : DareLib/Dare/getAPI_type  g_funcname=CanRx_0x281_BDC_TBOX_Req_PaSeatHeating  g_param=""  g_type=uint8  g_size=-1
      settings: AttributesFormatString=%<g_funcname>  SourceProductName=Dare Library
  VentAdj_PowerMode : DareLib/Dare/getAPI_type  g_funcname=Rte_GetVfb_PowerMode  g_param=""  g_type=uint8  g_enum=enPowerModeSts  g_size=-1
      settings: AttributesFormatString=%<g_funcname>  SourceProductName=Dare Library
  VentAdj_RecoverDefaultFlag : DareLib/Dare/getAPI_type  g_funcname=GetRecoverDefaultFlag  g_param=""  g_type=uint8  g_size=-1
      settings: AttributesFormatString=%<g_funcname>  SourceProductName=Dare Library
  VentAdj_RemoteModeFlag : DareLib/Dare/getAPI_type  g_funcname=Rte_GetVfb_RemoteModeFlag  g_param=""  g_type=uint8  g_size=-1
      settings: AttributesFormatString=%<g_funcname>  SourceProductName=Dare Library
  VentAdj_RunMaxTime : DareLib/Dare/getAPI_type  g_funcname=Srvl_GetMemIndexDataU8  g_param=EN_MemIndex_Vent_RunMaxTime  g_type=uint8  g_size=-1
      settings: AttributesFormatString=%<g_funcname>  SourceProductName=Dare Library
  VentAdj_ThirdCmdFaultSts : DareLib/Dare/getAPI_type  g_funcname=Rte_GetVfb_ThirdVentCmdFaultSts  g_param=""  g_type=uint8  g_enum=enVentCmdFault  g_size=-1
      settings: AttributesFormatString=%<g_funcname>  SourceProductName=Dare Library
  VentAdj_ThirdCmdFaultSts4DTC : DareLib/Dare/getAPI_type  g_funcname=Vfb_Reserved_0  g_param=""  g_type=uint8  g_enum=enVentCmdFault  g_size=-1
      settings: AttributesFormatString=%<g_funcname>  SourceProductName=Dare Library
  VentAdj_ThirdDiagCmd : DareLib/Dare/getAPI_type  g_funcname=Vfb_Reserved_0  g_param=""  g_type=uint8  g_enum=enVentIoCmdLvl  g_size=-1
      settings: AttributesFormatString=%<g_funcname>  SourceProductName=Dare Library
  VentAdj_ThirdEnableConfig : DareLib/Dare/getAPI_type  g_funcname=Rte_GetVfb_ThirdVentEnable  g_param=""  g_type=uint8  g_size=-1
      settings: AttributesFormatString=%<g_funcname>  SourceProductName=Dare Library
  VentAdj_ThirdHMI_VentMessage : DareLib/Dare/getAPI_type  g_funcname=Vfb_Reserved_0  g_param=""  g_type=uint8  g_size=-1
      settings: AttributesFormatString=%<g_funcname>  SourceProductName=Dare Library
  VentAdj_ThirdTbox_VentMessage : DareLib/Dare/getAPI_type  g_funcname=Vfb_Reserved_0  g_param=""  g_type=uint8  g_size=-1
      settings: AttributesFormatString=%<g_funcname>  SourceProductName=Dare Library
  "VentAdj_ThirdVentStopReason " : DareLib/Dare/getAPI_type  g_funcname=Rte_GetVfb_ThirdVentStopReason  g_param=""  g_type=uint8  g_enum=enVentStopReason  g_size=-1
      settings: AttributesFormatString=%<g_funcname>  SourceProductName=Dare Library
  VentAdj_Third_HMI_HeatMsg : DareLib/Dare/getAPI_type  g_funcname=CanRx_0x351_IVI_SwsHeatSw  g_param=""  g_type=uint8  g_size=-1
      settings: AttributesFormatString=%<g_funcname>  SourceProductName=Dare Library
  VentAdj_Third_Tbox_HeatMsg : DareLib/Dare/getAPI_type  g_funcname=CanRx_0x281_BDC_TBOX_Req_Steeringwheel_heating  g_param=""  g_type=uint8  g_size=-1
      settings: AttributesFormatString=%<g_funcname>  SourceProductName=Dare Library
  VentAdj_TimeOutPrm : DareLib/Dare/getAPI_type  g_funcname=Srvl_GetMemIndexDataU8  g_param=EN_MemIndex_Vent_TimeOutPrm  g_type=uint8  g_size=-1
      settings: AttributesFormatString=%<g_funcname>  SourceProductName=Dare Library
  VentAdj_VehicleRunFlag : DareLib/Dare/getAPI_type  g_funcname=Rte_GetVfb_VehicleRunFlag  g_param=""  g_type=uint8  g_size=-1
      settings: AttributesFormatString=%<g_funcname>  SourceProductName=Dare Library
  VentAdj_VentMsgLostFlag : DareLib/Dare/getAPI_type  g_funcname=Vfb_Reserved_0  g_param=""  g_type=uint8  g_size=-1
      settings: AttributesFormatString=%<g_funcname>  SourceProductName=Dare Library
  VentAdj_VoltMode : DareLib/Dare/getAPI_type  g_funcname=Rte_GetVfb_VoltMode  g_param=""  g_type=uint8  g_enum=enFinalPowerMode  g_size=-1
      settings: AttributesFormatString=%<g_funcname>  SourceProductName=Dare Library
  RTE_Signal : Outport
  wires:
  Bus Creator/1 -> RTE_Signal/1  "RTE_Signal"
  VentAdj_D_SimuIndex_DRVent/1 -> Bus Creator/1  "VentAdj_D_SimuIndex_DRVent"
  VentAdj_D_SimuIndex_PAVent/1 -> Bus Creator/2  "VentAdj_D_SimuIndex_PAVent"
  VentAdj_D_SimuIndex_ThirdVent/1 -> Bus Creator/3  "VentAdj_D_SimuIndex_ThirdVent"
  VentAdj_RemoteModeFlag/1 -> Bus Creator/4  "VentAdj_RemoteModeFlag"
  VentAdj_EngineRunFlag/1 -> Bus Creator/5  "VentAdj_EngineRunFlag"
  VentAdj_DriverCmdFaultSts/1 -> Bus Creator/6  "VentAdj_DriverCmdFaultSts"
  VentAdj_PasCmdFaultSts/1 -> Bus Creator/7  "VentAdj_PasCmdFaultSts"
  VentAdj_ThirdCmdFaultSts/1 -> Bus Creator/8  "VentAdj_ThirdCmdFaultSts"
  VentAdj_DrVentStopReason/1 -> Bus Creator/9  "VentAdj_DrVentStopReason"
  VentAdj_PaVentStopReason/1 -> Bus Creator/10  "VentAdj_PaVentStopReason"
  "VentAdj_ThirdVentStopReason "/1 -> Bus Creator/11  "VentAdj_ThirdVentStopReason"
  VentAdj_DrHeatFlg/1 -> Bus Creator/12  "VentAdj_DrHeatFlg"
  VentAdj_PaHeatFlg/1 -> Bus Creator/13  "VentAdj_PaHeatFlg"
  VentAdj_3rdHeatFlg/1 -> Bus Creator/14  "VentAdj_3rdHeatFlg"
  VentAdj_DriverCmdFaultSts4DTC/1 -> Bus Creator/15  "VentAdj_DriverCmdFaultSts4DTC"
  VentAdj_PasCmdFaultSts4DTC/1 -> Bus Creator/16  "VentAdj_PasCmdFaultSts4DTC"
  VentAdj_ThirdCmdFaultSts4DTC/1 -> Bus Creator/17  "VentAdj_ThirdCmdFaultSts4DTC"
  VentAdj_VehicleRunFlag/1 -> Bus Creator/18  "VentAdj_VehicleRunFlag"
  VentAdj_DriverHMI_VentMessage/1 -> Bus Creator/19  "VentAdj_DriverHMI_VentMessage"
  VentAdj_DriverTbox_VentMessage/1 -> Bus Creator/20  "VentAdj_DriverTbox_VentMessage"
  VentAdj_PassengerHMI_VentMessage/1 -> Bus Creator/21  "VentAdj_PassengerHMI_VentMessage"
  VentAdj_PassengerTbox_VentMessage/1 -> Bus Creator/22  "VentAdj_PassengerTbox_VentMessage"
  VentAdj_ThirdHMI_VentMessage/1 -> Bus Creator/23  "VentAdj_ThirdHMI_VentMessage"
  VentAdj_ThirdTbox_VentMessage/1 -> Bus Creator/24  "VentAdj_ThirdTbox_VentMessage"
  VentAdj_DriverDiagCmd/1 -> Bus Creator/25  "VentAdj_DriverDiagCmd"
  VentAdj_PassengerDiagCmd/1 -> Bus Creator/26  "VentAdj_PassengerDiagCmd"
  VentAdj_ThirdDiagCmd/1 -> Bus Creator/27  "VentAdj_ThirdDiagCmd"
  VentAdj_TimeOutPrm/1 -> Bus Creator/28  "VentAdj_TimeOutPrm"
  VentAdj_RunMaxTime/1 -> Bus Creator/29  "VentAdj_RunMaxTime"
  VentAdj_CarType/1 -> Bus Creator/30  "VentAdj_CarType"
  VentAdj_DriverEnableConfig/1 -> Bus Creator/31  "VentAdj_DriverEnableConfig"
  VentAdj_PassengerEnableConfig/1 -> Bus Creator/32  "VentAdj_PassengerEnableConfig"
  VentAdj_ThirdEnableConfig/1 -> Bus Creator/33  "VentAdj_ThirdEnableConfig"
  VentAdj_RecoverDefaultFlag/1 -> Bus Creator/34  "VentAdj_RecoverDefaultFlag"
  VentAdj_Driver_HMI_HeatMsg/1 -> Bus Creator/35  "VentAdj_Driver_HMI_HeatMsg"
  VentAdj_Driver_Tbox_HeatMsg/1 -> Bus Creator/36  "VentAdj_Driver_Tbox_HeatMsg"
  VentAdj_Passenger_HMI_HeatMsg/1 -> Bus Creator/37  "VentAdj_Passenger_HMI_HeatMsg"
  VentAdj_Passenger_Tbox_HeatMsg/1 -> Bus Creator/38  "VentAdj_Passenger_Tbox_HeatMsg"
  VentAdj_Third_HMI_HeatMsg/1 -> Bus Creator/39  "VentAdj_Third_HMI_HeatMsg"
  VentAdj_Third_Tbox_HeatMsg/1 -> Bus Creator/40  "VentAdj_Third_Tbox_HeatMsg"
  VentAdj_VentMsgLostFlag/1 -> Bus Creator/41  "VentAdj_VentMsgLostFlag"
  VentAdj_CanDrvVentLvl/1 -> Bus Creator/42  "VentAdj_CanDrvVentLvl"
  VentAdj_CanPasVentLvl/1 -> Bus Creator/43  "VentAdj_CanPasVentLvl"
  VentAdj_CanThirdVentLvl/1 -> Bus Creator/44  "VentAdj_CanThirdVentLvl"
  VentAdj_DrVentFlg/1 -> Bus Creator/45  "VentAdj_DrVentFlg"
  VentAdj_PaVentFlg/1 -> Bus Creator/46  "VentAdj_PaVentFlg"
  VentAdj_PowerMode/1 -> Bus Creator/47  "VentAdj_PowerMode"
  VentAdj_VoltMode/1 -> Bus Creator/48  "VentAdj_VoltMode"

== system Appl_VentAdj_CtrlModel/LogicCtrl/LocalAdjustCtrl/LimitDeal/DiagnoseFunction ==
  DiagCommand : Inport
  InLevel : Inport  Port=2
  CurrentType : Inport  Port=3
  f : TriggerPort  TriggerType=function-call  VariantControl=(inherit)
      settings: CopyFcn=Stateflow.SLINSF.SimulinkMan.removeBlockPreDeleteFcn  PreDeleteFcn=Stateflow.SLINSF.SimulinkMan.unsafePredeleteFcn
  Diagnose : Stateflow chart  TreatAsAtomicUnit=on
  Level : Outport
  Type : Outport  Port=2
  wires:
  DiagCommand/1 -> Diagnose/1(DiagCommand)
  InLevel/1 -> Diagnose/2(InLevel)
  CurrentType/1 -> Diagnose/3(CurrentType)
  Diagnose/1(Level) -> Level/1
  Diagnose/2(Type) -> Type/1

== system Appl_VentAdj_CtrlModel/LogicCtrl/LocalAdjustCtrl/LimitDeal/DiagnoseFunction1 ==
  DiagCommand : Inport
  InLevel : Inport  Port=2
  CurrentType : Inport  Port=3
  f : TriggerPort  TriggerType=function-call  VariantControl=(inherit)
      settings: CopyFcn=Stateflow.SLINSF.SimulinkMan.removeBlockPreDeleteFcn  PreDeleteFcn=Stateflow.SLINSF.SimulinkMan.unsafePredeleteFcn
  Diagnose : Stateflow chart  TreatAsAtomicUnit=on
  Level : Outport
  Type : Outport  Port=2
  wires:
  DiagCommand/1 -> Diagnose/1(DiagCommand)
  InLevel/1 -> Diagnose/2(InLevel)
  CurrentType/1 -> Diagnose/3(CurrentType)
  Diagnose/1(Level) -> Level/1
  Diagnose/2(Type) -> Type/1

== system Appl_VentAdj_CtrlModel/LogicCtrl/LocalAdjustCtrl/LimitDeal/DiagnoseFunction2 ==
  DiagCommand : Inport
  InLevel : Inport  Port=2
  CurrentType : Inport  Port=3
  f : TriggerPort  TriggerType=function-call  VariantControl=(inherit)
      settings: CopyFcn=Stateflow.SLINSF.SimulinkMan.removeBlockPreDeleteFcn  PreDeleteFcn=Stateflow.SLINSF.SimulinkMan.unsafePredeleteFcn
  Diagnose : Stateflow chart  TreatAsAtomicUnit=on
  Level : Outport
  Type : Outport  Port=2
  wires:
  DiagCommand/1 -> Diagnose/1(DiagCommand)
  InLevel/1 -> Diagnose/2(InLevel)
  CurrentType/1 -> Diagnose/3(CurrentType)
  Diagnose/1(Level) -> Level/1
  Diagnose/2(Type) -> Type/1

== system Appl_VentAdj_CtrlModel/LogicCtrl/LocalAdjustCtrl/LimitDeal/LevelLimitFunction ==
  OriginalLevel : Inport
  Error : Inport  Port=2
  OppositeCmd : Inport  Port=3
  CarType : Inport  Port=4
  Vent_CanMessageLostFlag : Inport  Port=5
  Vent_RecoverDefaultFlag : Inport  Port=6
  f : TriggerPort  TriggerType=function-call  VariantControl=(inherit)
      settings: CopyFcn=Stateflow.SLINSF.SimulinkMan.removeBlockPreDeleteFcn  PreDeleteFcn=Stateflow.SLINSF.SimulinkMan.unsafePredeleteFcn
  LevelLimit : Stateflow chart  TreatAsAtomicUnit=on
  Level : Outport
  StopReason : Outport  Port=2
  wires:
  OriginalLevel/1 -> LevelLimit/1(OriginalLevel)
  Error/1 -> LevelLimit/2(Error)
  CarType/1 -> LevelLimit/3(CarType)
  OppositeCmd/1 -> LevelLimit/4(OppositeCmd)
  Vent_CanMessageLostFlag/1 -> LevelLimit/5(Vent_CanMessageLostFlag)
  Vent_RecoverDefaultFlag/1 -> LevelLimit/6(Vent_RecoverDefaultFlag)
  LevelLimit/1(Level) -> Level/1
  LevelLimit/2(StopReason) -> StopReason/1

== system Appl_VentAdj_CtrlModel/LogicCtrl/LocalAdjustCtrl/LimitDeal/LevelLimitFunction1 ==
  OriginalLevel : Inport
  Error : Inport  Port=2
  OppositeCmd : Inport  Port=3
  CarType : Inport  Port=4
  Vent_CanMessageLostFlag : Inport  Port=5
  Vent_RecoverDefaultFlag : Inport  Port=6
  f : TriggerPort  TriggerType=function-call  VariantControl=(inherit)
      settings: CopyFcn=Stateflow.SLINSF.SimulinkMan.removeBlockPreDeleteFcn  PreDeleteFcn=Stateflow.SLINSF.SimulinkMan.unsafePredeleteFcn
  LevelLimit : Stateflow chart  TreatAsAtomicUnit=on
  Level : Outport
  StopReason : Outport  Port=2
  wires:
  OriginalLevel/1 -> LevelLimit/1(OriginalLevel)
  Error/1 -> LevelLimit/2(Error)
  CarType/1 -> LevelLimit/3(CarType)
  OppositeCmd/1 -> LevelLimit/4(OppositeCmd)
  Vent_CanMessageLostFlag/1 -> LevelLimit/5(Vent_CanMessageLostFlag)
  Vent_RecoverDefaultFlag/1 -> LevelLimit/6(Vent_RecoverDefaultFlag)
  LevelLimit/1(Level) -> Level/1
  LevelLimit/2(StopReason) -> StopReason/1
